simulink model "SimpleBot_V4"  (R2024a)
settings: Solver=VariableStepAuto  StartTime=0.0  StopTime=1.5  FixedStep=0.01  RelTol=1e-3
values from neighbouring files (symbols this model uses):
  Achsabstand = 0.15    [Model1Sensibilities.m]    (also in Model1numericalPSA.m; Model2Sensibilities.m; Modellvalidierung.m; MotorSens2.m)
  B_dis = 0.25    [Model1Sensibilities.m]    (also in Model1numericalPSA.m = 0.15; Model2Sensibilities.m; Modellvalidierung.m = 0.15; MotorSens2.m)
  c_pose = [0 0 0 0 1 0 0 ... (first row only)    [Model2Sensibilities.m]    (also in ParamsModell.m; ParamsModell2.m; model1Sensibiliaet.m; robotmodel2Sensibilities.m)
  g = 9.81    [Model1Sensibilities.m]    (also in Model1numericalPSA.m; Model2Sensibilities.m; Modellvalidierung.m; MotorSens2.m)
  I_Bot = 0.0072    [Model1Sensibilities.m]    (also in Model1numericalPSA.m; Model2Sensibilities.m; Modellvalidierung.m; MotorSens2.m)
  I_Reifen = 1.8 * 10^-5    (= 1.8e-05)    [Model1Sensibilities.m]    (also in Model1numericalPSA.m; Model2Sensibilities.m; Modellvalidierung.m; ParamsModell.m)
  L_B = 0.12    [Model1numericalPSA.m]    (also in Modellvalidierung.m; ParamsModell.m; Sensitivitaetsanalyse.m; model1Sensibiliaet.m)
  m_ges = 1    [Model1Sensibilities.m]    (also in Model1numericalPSA.m; Model2Sensibilities.m; Modellvalidierung.m; MotorSens2.m)
  motor_BackEMFkoef = 0.0035    [Model1Sensibilities.m]    (also in Model1numericalPSA.m; Model2Sensibilities.m; Modellvalidierung.m; MotorSens2.m)
  motor_Daempfung = 9.12 * 10^-8    (= 9.12e-08)    [Model1Sensibilities.m]    (also in Model1numericalPSA.m; Model2Sensibilities.m; Modellvalidierung.m; MotorSens2.m)
  motor_Drehmomentkoef = 0.0174    [Model1Sensibilities.m]    (also in Model1numericalPSA.m = 0.0035; Model2Sensibilities.m; Modellvalidierung.m = 0.0035; MotorSens2.m)
  motor_Induktivitaet = 0.0002    [Model1Sensibilities.m]    (also in Model1numericalPSA.m; Model2Sensibilities.m; Modellvalidierung.m; MotorSens2.m)
  motor_traegheit = 0.847 * 10^-6    (= 8.47e-07)    [Model1Sensibilities.m]    (also in Model1numericalPSA.m; Model2Sensibilities.m; Modellvalidierung.m; MotorSens2.m)
  motor_Widerstand = 13.33    [Model1Sensibilities.m]    (also in Model1numericalPSA.m; Model2Sensibilities.m; Modellvalidierung.m; MotorSens2.m)
  Motoruebersetzung = 100    [Model1Sensibilities.m]    (also in Model1numericalPSA.m; Model2Sensibilities.m; Modellvalidierung.m; MotorSens2.m)
  mue_g = 0.1    [Model1Sensibilities.m]    (also in Model1numericalPSA.m; Model2Sensibilities.m; Modellvalidierung.m; MotorSens2.m)
  Reifen_Radius = 0.04    [Model1Sensibilities.m]    (also in Model1numericalPSA.m; Model2Sensibilities.m; Modellvalidierung.m; MotorSens2.m)
  x0s = [0 ... (first row only)    [Model2Sensibilities.m]    (also in MotorSens2.m = [; Motor_Sensitivitaet.m = [; Parameter.m = [; ParamsModell.m)
  Xi = 2/3    (= 0.666666666667)    [Model1Sensibilities.m]    (also in Model1numericalPSA.m = 0.333333333333; Model2Sensibilities.m; Modellvalidierung.m = 0.333333333333; MotorSens2.m)
  Zielpunkt = [1;1.2]    [Model2Sensibilities.m]    (also in MotorSens2.m; Motor_Sensitivitaet.m; Parameter.m; ParamsModell.m)
libraries: slpidlib x2, simulink x1, mobileRoboticsLib x1
settings Model: Creator=jakob  LastModifiedBy=jakob

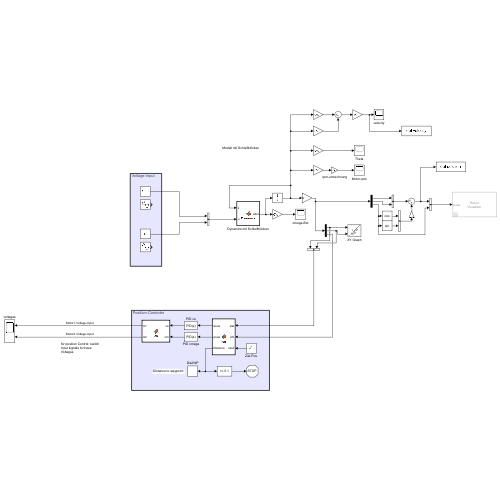
[thumbnail: Simulink's stored preview of the top-level diagram]
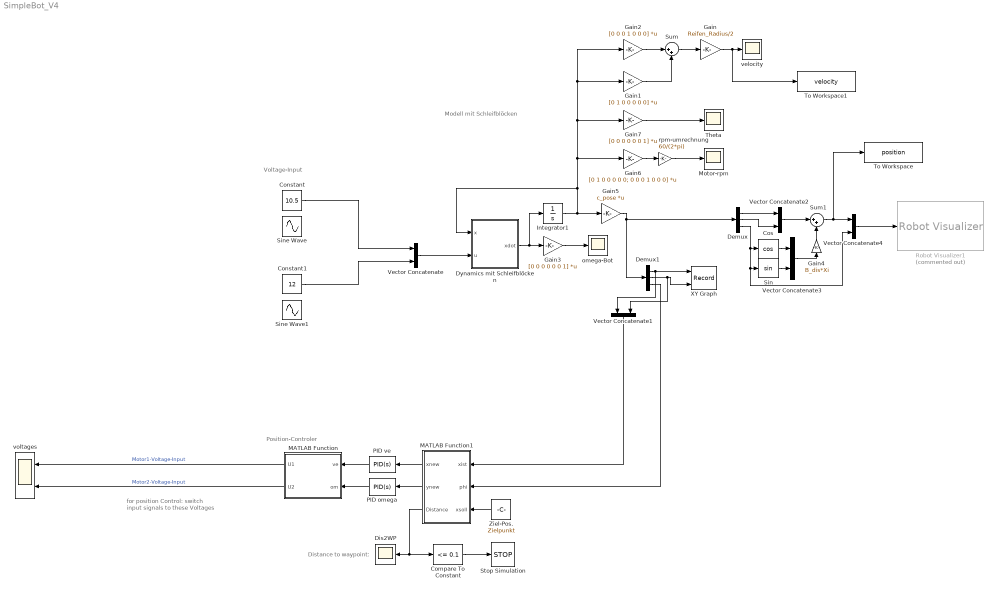
== system SimpleBot_V4 ==
  note: Modell mit Schleifblöcken
  note: Voltage-Input
  note: Distance to waypoint:
  note: for position Control: switch input signals to these Voltages
  note: Position-Controler
  Compare To Constant : simulink/Logic and Bit Operations/Compare To Constant  relop=<=  const=0.1  OutDataTypeStr=boolean
  Constant : Constant  Value=10.5  SampleTime=1
  Constant1 : Constant  Value=12  SampleTime=1
  Cos : Trigonometry  Operator=cos
  Demux : Demux  Outputs=3
  Demux1 : Demux  Outputs=3
  Dis2WP : Scope
  Dynamics mit Schleifblöcken : MATLAB Function  TreatAsAtomicUnit=on
  Gain : Gain  Gain=Reifen_Radius/2
  Gain1 : Gain  Gain=[0 1 0 0 0 0 0]  Multiplication=Matrix(K*u)
  Gain2 : Gain  Gain=[0 0 0 1 0 0 0]  Multiplication=Matrix(K*u)
  Gain3 : Gain  Gain=[0 0 0 0 0 0 1]  Multiplication=Matrix(K*u)
  Gain4 : Gain  Gain=B_dis*Xi
  Gain5 : Gain  Gain=c_pose  Multiplication=Matrix(K*u)
  Gain6 : Gain  Gain=[0 1 0 0 0 0 0; 0 0 0 1 0 0 0]  Multiplication=Matrix(K*u)
  Gain7 : Gain  Gain=[0 0 0 0 0 0 1]  Multiplication=Matrix(K*u)
  Integrator1 : Integrator  InitialCondition=x0s
  MATLAB Function : MATLAB Function  TreatAsAtomicUnit=on
  MATLAB Function1 : MATLAB Function  TreatAsAtomicUnit=on
  Motor-rpm : Scope
  PID omega : slpidlib/PID Controller  Controller=PID  Form=Parallel  TimeDomain=Continuous-time  UseExternalTs=off  SampleTime=-1  IntegratorMethod=Forward Euler  FilterMethod=Forward Euler  ControllerParametersSource=internal  P=-0.000440133321900821  I=-0.000927517880143504  UseKiTs=off  D=-4.71719040183482e-05  UseExternalDerivativeSource=off  N=66.1016813449342  UseFilter=on  TunerSelectOption=Transfer Function Based (PID Tuner App)  InitialConditionSource=internal  InitialConditionForIntegrator=0  InitialConditionForFilter=0  DifferentiatorICPrevScaledInput=0  ExternalReset=none  TrackingMode=off  Kt=1  LimitOutput=off  SatLimitsSource=internal  UpperSaturationLimit=inf  LowerSaturationLimit=-inf  LinearizeAsGain=on  AntiWindupMode=none  Kb=1  LimitIntegrator=off  UpperIntegratorSaturationLimit=inf  LowerIntegratorSaturationLimit=-inf  POutMin=[]  POutMax=[]  IOutMin=[]  IOutMax=[]  DOutMin=[]  DOutMax=[]  NOutMin=[]  NOutMax=[]  SumOutMin=[]  SumOutMax=[]  SaturationOutMin=[]  SaturationOutMax=[]  PParamMin=[]  PParamMax=[]  IParamMin=[]  IParamMax=[]  DParamMin=[]  DParamMax=[]  NParamMin=[]  NParamMax=[]  KbParamMin=[]  KbParamMax=[]  KtParamMin=[]  KtParamMax=[]  KbOutMin=[]  KbOutMax=[]  KtOutMin=[]  KtOutMax=[]  IntegratorOutMin=[]  IntegratorOutMax=[]  FilterOutMin=[]  FilterOutMax=[]  SumI1OutMin=[]  SumI1OutMax=[]  SumI2OutMin=[]  SumI2OutMax=[]  SumI3OutMin=[]  SumI3OutMax=[]  SumI4OutMin=[]  SumI4OutMax=[]  SumDOutMin=[]  SumDOutMax=[]  DifferentiatorOutMin=[]  DifferentiatorOutMax=[]  FilterDiffOutCoefMin=[]  FilterDiffOutCoefMax=[]  ReciprocalOutMin=[]  ReciprocalOutMax=[]  SumDenOutMin=[]  SumDenOutMax=[]  SumNumOutMin=[]  SumNumOutMax=[]  DivideOutMin=[]  DivideOutMax=[]  UdiffTsProdOutMin=[]  UdiffTsProdOutMax=[]  NTsProdOutMin=[]  NTsProdOutMax=[]  UintegralTsProdOutMin=[]  UintegralTsProdOutMax=[]  UngainTsProdOutMin=[]  UngainTsProdOutMax=[]  ClampingZeroOutDataTypeStr=Inherit: Inherit via back propagation  ClampingZeroOutMin=[]  ClampingZeroOutMax=[]  FilterDenConstantOutDataTypeStr=Inherit: Inherit via back propagation  FilterDenConstantOutMin=[]  FilterDenConstantOutMax=[]  PCopyOutDataTypeStr=Inherit: Inherit via back propagation  PCopyOutMin=[]  PCopyOutMax=[]  NCopyOutDataTypeStr=Inherit: Inherit via back propagation  NCopyOutMin=[]  NCopyOutMax=[]  IntegratorContinuousStateAttributes=''  IntegratorStateMustResolveToSignalObject=off  IntegratorRTWStateStorageClass=Auto  FilterContinuousStateAttributes=''  FilterStateMustResolveToSignalObject=off  FilterRTWStateStorageClass=Auto  ParallelPVariant=InternalParameters  IdealPVariant=Disabled  IVariant=InternalParameters  DVariant=InternalParameters  IntegratorVariant=Continuous  SatVariant=Disabled  AWVariant=Passthrough  PCopyVariant=Disabled  TRVariant=Disabled  FdbkBlocksVariant=Forward  IdealPFdbkVariant=Disabled  SatFdbkVariant=Disabled  DerivativeFilterVariant=ContFilter  NVariant=InternalParameters  NCopyVariant=Disabled  FilterICVariant=InternalICsFilter  IntegratorICVariant=InternalICs  ExternalResetVariant=Disabled  TRSumVariant=Passthrough  SumFdbkVariant=Disabled  SumVariant=Sum_PID  TsampFilterVariant=InternalTs  TsampNgainVariant=Passthrough  TsampIntegralVariant=Disabled_SignalSpec  ExternalSaturationOutDataTypeStr=Inherit: Same as second input  DerivativeSourceVariant=ErrorSignal
  PID ve : slpidlib/PID Controller  Controller=PID  Form=Parallel  TimeDomain=Continuous-time  UseExternalTs=off  SampleTime=-1  IntegratorMethod=Forward Euler  FilterMethod=Forward Euler  ControllerParametersSource=internal  P=-4.08143923597295e-05  I=-2.0321677011973e-05  UseKiTs=off  D=-8.15536700886172e-06  UseExternalDerivativeSource=off  N=349.581689357537  UseFilter=on  TunerSelectOption=Transfer Function Based (PID Tuner App)  InitialConditionSource=internal  InitialConditionForIntegrator=0  InitialConditionForFilter=0  DifferentiatorICPrevScaledInput=0  ExternalReset=none  TrackingMode=off  Kt=1  LimitOutput=off  SatLimitsSource=internal  UpperSaturationLimit=inf  LowerSaturationLimit=-inf  LinearizeAsGain=on  AntiWindupMode=none  Kb=1  LimitIntegrator=off  UpperIntegratorSaturationLimit=inf  LowerIntegratorSaturationLimit=-inf  POutMin=[]  POutMax=[]  IOutMin=[]  IOutMax=[]  DOutMin=[]  DOutMax=[]  NOutMin=[]  NOutMax=[]  SumOutMin=[]  SumOutMax=[]  SaturationOutMin=[]  SaturationOutMax=[]  PParamMin=[]  PParamMax=[]  IParamMin=[]  IParamMax=[]  DParamMin=[]  DParamMax=[]  NParamMin=[]  NParamMax=[]  KbParamMin=[]  KbParamMax=[]  KtParamMin=[]  KtParamMax=[]  KbOutMin=[]  KbOutMax=[]  KtOutMin=[]  KtOutMax=[]  IntegratorOutMin=[]  IntegratorOutMax=[]  FilterOutMin=[]  FilterOutMax=[]  SumI1OutMin=[]  SumI1OutMax=[]  SumI2OutMin=[]  SumI2OutMax=[]  SumI3OutMin=[]  SumI3OutMax=[]  SumI4OutMin=[]  SumI4OutMax=[]  SumDOutMin=[]  SumDOutMax=[]  DifferentiatorOutMin=[]  DifferentiatorOutMax=[]  FilterDiffOutCoefMin=[]  FilterDiffOutCoefMax=[]  ReciprocalOutMin=[]  ReciprocalOutMax=[]  SumDenOutMin=[]  SumDenOutMax=[]  SumNumOutMin=[]  SumNumOutMax=[]  DivideOutMin=[]  DivideOutMax=[]  UdiffTsProdOutMin=[]  UdiffTsProdOutMax=[]  NTsProdOutMin=[]  NTsProdOutMax=[]  UintegralTsProdOutMin=[]  UintegralTsProdOutMax=[]  UngainTsProdOutMin=[]  UngainTsProdOutMax=[]  ClampingZeroOutDataTypeStr=Inherit: Inherit via back propagation  ClampingZeroOutMin=[]  ClampingZeroOutMax=[]  FilterDenConstantOutDataTypeStr=Inherit: Inherit via back propagation  FilterDenConstantOutMin=[]  FilterDenConstantOutMax=[]  PCopyOutDataTypeStr=Inherit: Inherit via back propagation  PCopyOutMin=[]  PCopyOutMax=[]  NCopyOutDataTypeStr=Inherit: Inherit via back propagation  NCopyOutMin=[]  NCopyOutMax=[]  IntegratorContinuousStateAttributes=''  IntegratorStateMustResolveToSignalObject=off  IntegratorRTWStateStorageClass=Auto  FilterContinuousStateAttributes=''  FilterStateMustResolveToSignalObject=off  FilterRTWStateStorageClass=Auto  ParallelPVariant=InternalParameters  IdealPVariant=Disabled  IVariant=InternalParameters  DVariant=InternalParameters  IntegratorVariant=Continuous  SatVariant=Disabled  AWVariant=Passthrough  PCopyVariant=Disabled  TRVariant=Disabled  FdbkBlocksVariant=Forward  IdealPFdbkVariant=Disabled  SatFdbkVariant=Disabled  DerivativeFilterVariant=ContFilter  NVariant=InternalParameters  NCopyVariant=Disabled  FilterICVariant=InternalICsFilter  IntegratorICVariant=InternalICs  ExternalResetVariant=Disabled  TRSumVariant=Passthrough  SumFdbkVariant=Disabled  SumVariant=Sum_PID  TsampFilterVariant=InternalTs  TsampNgainVariant=Passthrough  TsampIntegralVariant=Disabled_SignalSpec  ExternalSaturationOutDataTypeStr=Inherit: Same as second input  DerivativeSourceVariant=ErrorSignal
  Robot Visualizer1 : mobileRoboticsLib/Environments/Robot Visualizer  Commented=on  robotRadius=0.15  mapName=myMap  showTrajectory=on  hasWaypoints=off  hasLidar=off  sensorOffset=[ 0, 0 ]  scanAngles=[ -pi/4, 0, pi/4 ]  hasObjDetector=off  objDetectorOffset=[ 0, 0 ]  objDetectorAngle=0  objDetectorFOV=pi/4  objDetectorMaxRange=5  objectColors=[ 1, 0, 0; 0, 1, 0; 0, 0, 1 ]  objectMarkers=s
  Sin : Trigonometry
  Sine Wave : Sin  Amplitude=4  Bias=8  Frequency=2  SampleTime=0
  Sine Wave1 : Sin  Amplitude=4  Bias=8  Frequency=3  SampleTime=0
  Stop Simulation : Stop
  Sum : Sum  Inputs=|++
  Sum1 : Sum  Inputs=|++
  Theta : Scope
  To Workspace : ToWorkspace  VariableName=position  SaveFormat=Timeseries  SampleTime=-1
  To Workspace1 : ToWorkspace  VariableName=velocity  SaveFormat=Structure With Time  SampleTime=-1
  Vector Concatenate{,1..4} (5 alike) : Concatenate
  XY Graph : Record  FileSettingsInternal="{\"entries\":[{\"content\":{\"excelSettings\":{\"content\":{},\"type\":\"Streamout.ExcelSettings\"}},\"type\":\"Streamout.FileSettingStorage\",\"uuid\":\"\"}],\"packageUris\":[\"http:\\/\\/schema.mathworks.com\\/mf0\\/streamout_blocks\\/R2020a\"],\"version\":\"1.0\"}"  Layout=[1 1]  SignalsInternal="{\"entries\":[{\"content\":{\"signals\":[{\"content\":{\"blockPath\":[],\"dimensions\":[1,1],\"domain\":\"\",\"lineColor\":\"#64d413\",\"lineWidth\":2,\"plots\":[ 1 ],\"port\":1,\"sid\":[\"\"],\"signalID\":1,\"signalName\":\"Demux1:1\"},\"type\":\"RecordBlkView.Signal\",\"uuid\":\"\"},{\"content\":{\"blockPath\":[],\"dimensions\":[1,1],\"domain\":\"\",\"lineColor\":\"#ff13a6\",\"lineWidth\":2,\"plots\":[ 1 ],\"port\":2,\"sid\":[\"\"],\"signalID\":2,\"signalName\":\"Demux1:2\"},\"type\":\"RecordBlkView.Signal\",\"uuid\":\"\"}]},\"type\":\"RecordBlkView.InputSignals\",\"uuid\":\"\"}],\"packageUris\":[\"http:\\/\\/schema.mathworks.com\\/mf0\\/streamout_blocks\\/R2020a\"],\"version\":\"1.0\"}"  VisualizationBindings="{\"xyplotplugin\":{\"info\":[{\"series\":[{\"bindingParametersList\":[{\"parameter\":\"X-Axis\",\"signalID\":1,\"signalName\":\"Demux1:1\"},{\"parameter\":\"Y-Axis\",\"signalID\":2,\"signalName\":\"Demux1:2\"}],\"seriesID\":0}],\"subplotID\":1}]}}"  CompatibilityTag=XY
  Ziel-Pos. : Constant  Value=Zielpunkt
  omega-Bot : Scope
  rpm-umrechnung : Gain  Gain=60/(2*pi)
  velocity : Scope
  voltages : Scope  NumInputPorts=2
  wires:
  Gain6/1 -> rpm-umrechnung/1
  Gain7/1 -> Theta/1
  rpm-umrechnung/1 -> Motor-rpm/1
  Sum/1 -> Gain/1
  Vector Concatenate/1 -> Dynamics mit Schleifblöcken/2(u)
  Gain1/1 -> Sum/2
  Integrator1/1 -> Gain6/1, Gain2/1, Gain1/1, Gain7/1, Dynamics mit Schleifblöcken/1(x), Gain5/1
  Gain2/1 -> Sum/1
  Demux1/1 -> XY Graph/1, Vector Concatenate1/1
  Demux1/2 -> Vector Concatenate1/2, XY Graph/2
  Gain/1 -> To Workspace1/1, velocity/1
  Dynamics mit Schleifblöcken/1(xdot) -> Integrator1/1, Gain3/1
  MATLAB Function1/3(Distance) -> Compare To Constant/1, Dis2WP/1
  MATLAB Function1/1(xnew) -> PID ve/1
  MATLAB Function/1(U1) -> voltages/1  "Motor1-Voltage-Input"
  Demux1/3 -> MATLAB Function1/2(phi)
  Ziel-Pos./1 -> MATLAB Function1/3(xsoll)
  MATLAB Function/2(U2) -> voltages/2  "Motor2-Voltage-Input"
  Compare To Constant/1 -> Stop Simulation/1
  MATLAB Function1/2(ynew) -> PID omega/1
  Vector Concatenate1/1 -> MATLAB Function1/1(xist)
  PID ve/1 -> MATLAB Function/1(ve)
  PID omega/1 -> MATLAB Function/2(om)
  Constant/1 -> Vector Concatenate/1
  Constant1/1 -> Vector Concatenate/2
  Demux/1 -> Vector Concatenate2/1
  Demux/3 -> Vector Concatenate4/2, Sin/1, Cos/1
  Gain4/1 -> Sum1/2
  Vector Concatenate2/1 -> Sum1/1
  Vector Concatenate4/1 -> Robot Visualizer1/1
  Cos/1 -> Vector Concatenate3/1
  Vector Concatenate3/1 -> Gain4/1
  Sum1/1 -> To Workspace/1, Vector Concatenate4/1
  Gain5/1 -> Demux/1, Demux1/1
  Demux/2 -> Vector Concatenate2/2
  Sin/1 -> Vector Concatenate3/2
  Gain3/1 -> omega-Bot/1

== matlab function SimpleBot_V4/MATLAB Function ==
  data: U1 output; U2 output; ve input; om input; motor_BackEMFkoef parameter; Motoruebersetzung parameter; Achsabstand parameter; Reifen_Radius parameter
function [U1, U2] = fcn(ve, om,motor_BackEMFkoef, Motoruebersetzung, Achsabstand, Reifen_Radius)

U1 = (Motoruebersetzung / motor_BackEMFkoef) * ((ve-om*(Achsabstand/2))/Reifen_Radius);
U2 = (Motoruebersetzung / motor_BackEMFkoef) * ((ve+om*(Achsabstand/2))/Reifen_Radius);

% U1 = max(min(U1, 60), -60);
% U2 = max(min(U2, 60), -60);

== matlab function SimpleBot_V4/Dynamics mit Schleifblöcken ==
  data: x input; u input; xdot output; Motoruebersetzung parameter; motor_traegheit parameter; m_ges parameter; Reifen_Radius parameter; I_Bot parameter; Achsabstand parameter; motor_Drehmomentkoef parameter; motor_Daempfung parameter; motor_Widerstand parameter; motor_Induktivitaet parameter; motor_BackEMFkoef parameter; mue_g parameter; g parameter; Xi parameter; B_dis parameter; I_Reifen parameter; L_B parameter
function xdot = Dynamics(x,u,Motoruebersetzung, motor_traegheit, m_ges, Reifen_Radius, I_Bot, Achsabstand, motor_Drehmomentkoef, motor_Daempfung,motor_Widerstand, motor_Induktivitaet, motor_BackEMFkoef,mue_g, g, Xi, B_dis,I_Reifen,L_B)

%% Input
%x-vec:
i_m1 = x(1);
om_m1 = x(2);
i_m2 = x(3);
om_m2 = x(4);
theta = x(7);

%Spannungs-Eingang
Ue1 = u(1);
Ue2 = u(2);

%% Träheitstensor
J_Mn = Motoruebersetzung^2 * motor_traegheit;
C1 = (m_ges*Reifen_Radius^2)/4 - (I_Bot*Reifen_Radius^2)/(Achsabstand^2);
C2 = (m_ges*Reifen_Radius^2)/4 + (I_Bot*Reifen_Radius^2)/(Achsabstand^2);

M11 = J_Mn + C1 + I_Reifen;
M12 = C2;
M21 = M12;
M22 = M11;

J_g = [M11 M12;
       M21 M22];


%% Berechnung der Belastungen
% Grenzgeschwindigkeit gegen 0
v_Tresh = 1e-3;
% Grenzwinkelgeschwindigkeit gegen 0
omega_Tresh = 1e-3;
% Grenzwinkelgeschwindigkeits-Unterschied
eps_om = 1e-6;
% Steigungen für Glättungsfunktionen
k_smooth = 5000;
k_xppos = 100;
k_xp = 5 / eps_om;
% konstante Nenner-Erwiterungen für Singlaritäten
delta_sig_sq = 1e-6;
xp_delta = 1e-6;
eta_abs_sq = (eps_om/10)^2;

% Angriffspunkte der Reibngskräfte
B1 = [(1-Xi)*B_dis; L_B/2];
B2 = [(1-Xi)*B_dis; -L_B/2];

% Berechnung der reibungskraft-Angriffswinkel über Ermittlung von
% Geschwindigkeitspol xp
OmegaSum = om_m1 + om_m2;
deltaOmega = om_m2-om_m1;
smooth_abs_DeltaOmega = sqrt(deltaOmega^2 + eta_abs_sq);

v_Bot = (Reifen_Radius/2)*OmegaSum;
omega_Bot = (Reifen_Radius/Achsabstand)*smooth_abs_DeltaOmega;

% Glättungsfunktionen für Reibungskraft-> keine Reibung bei v_Bot / omega_Bot =0
smooth_factor_straight = 0.5 * (1 + tanh(k_smooth * (v_Bot - v_Tresh)));
smooth_factor_spin = 0.5 * (1 + tanh(k_smooth * (omega_Bot - omega_Tresh)));
C_Frb = mue_g * m_ges * g * (Xi/2);
Frb_smooth_straight = smooth_factor_straight * C_Frb;
Frb_smooth_spin = smooth_factor_spin * C_Frb;

% Bestimmung von Geschwndigkeitspol xp
w = 0.5 * (1 + tanh(k_xp*(smooth_abs_DeltaOmega - eps_om)));

inv_xp_A_const = 1e-6;

inv_xp_B_turn_nun = (2/Achsabstand) * deltaOmega * OmegaSum;
inv_xp_B_turn_dun = OmegaSum^2 + delta_sig_sq;
inv_xp_B_turn = inv_xp_B_turn_nun / inv_xp_B_turn_dun;

inv_xp_smooth = (1-w) * inv_xp_A_const + w * inv_xp_B_turn;
xp_smooth = 1./(inv_xp_smooth+xp_delta);

xppos_translation = [-Xi*B_dis; xp_smooth];
xppos_turnonpint = [-Xi*B_dis; 0];

s = 1- tanh((k_xppos * OmegaSum)^2);
xppos = (1-s)* xppos_translation + s * xppos_turnonpint;

% Bestimmung von angriffswinkel von Reibkräften
B1xp = xppos - B1;
B2xp = xppos - B2;
Fb1_dir = [B1xp(2);-B1xp(1)];
Fb2_dir = [B2xp(2);-B2xp(1)];
Fb1_dir_unit = Fb1_dir / norm(Fb1_dir);
Fb2_dir_unit = Fb2_dir / norm(Fb2_dir);
FRB1spin = Frb_smooth_spin * Fb1_dir_unit;
FRB2spin = Frb_smooth_spin * Fb2_dir_unit;

% Durch reibungskräfte resultierende Momente am Roboter
M_FR1v = cross([B1;0],[FRB1spin;0]);
M_FR1 = M_FR1v(3);
M_FR2v = cross([B2;0],[FRB2spin;0]);
M_FR2 = M_FR2v(3);

% Gesamte Momenten-Belastung aufgrund der reibung bei Kontaktpunkten
Tr1_smooth = -(Frb_smooth_straight* Reifen_Radius/2) * (Fb1_dir_unit(1) + Fb2_dir_unit(1)) + w*(Reifen_Radius/Achsabstand)*(M_FR1+M_FR2);
Tr2_smooth = -(Frb_smooth_straight* Reifen_Radius/2) * (Fb1_dir_unit(1) + Fb2_dir_unit(1)) - w*(Reifen_Radius/Achsabstand)*(M_FR1+M_FR2);

% Gesamte Belastungen an den Motoren
M_belastungen = [Motoruebersetzung * motor_Drehmomentkoef * i_m1 - Motoruebersetzung^2 * motor_Daempfung*om_m1 + Tr1_smooth;
                 Motoruebersetzung * motor_Drehmomentkoef * i_m2 - Motoruebersetzung^2 * motor_Daempfung*om_m2 + Tr2_smooth];

% Bestimmung von Winkelbeschleunigungen der Motoren
om_dot = J_g \ M_belastungen;

%% Aufstellen von x-dot
di1dt = -(motor_Widerstand/motor_Induktivitaet) * i_m1 - (Motoruebersetzung * motor_BackEMFkoef/motor_Induktivitaet) * om_m1 + (1/motor_Induktivitaet)* Ue1;
dom1dt = om_dot(1);
di2dt = -(motor_Widerstand/motor_Induktivitaet) * i_m2 - (Motoruebersetzung * motor_BackEMFkoef/motor_Induktivitaet) * om_m2 + (1/motor_Induktivitaet)* Ue2;
dom2dt = om_dot(2);
vx = (Reifen_Radius/2) * (om_m1 + om_m2) * cos(theta);
vy = (Reifen_Radius/2) * (om_m1 + om_m2) * sin(theta);
dthetadt = (Reifen_Radius/Achsabstand) * (om_m2-om_m1);

xdot = [di1dt;dom1dt;di2dt;dom2dt;vx;vy;dthetadt];

== matlab function SimpleBot_V4/MATLAB Function1 ==
  data: xist input; phi input; xnew output; xsoll input; ynew output; Distance output
function [xnew,ynew, Distance] = fcn(xist,phi,xsoll)

Pos_Error = xist-xsoll;   %Distance to waypoint in global coordinates      

RotPhi = [cos(phi) +sin(phi);-sin(phi) cos(phi)];

E_bot = RotPhi * Pos_Error;
xnew = E_bot(1);        %direct distance to waypoint (on body coordinates)
ynew = E_bot(2);        %lateral distance to waypoint (on body coordinates)

Distance = norm(Pos_Error);
